simulink model "hot_region_scheduler"  (R2021a)
settings: Solver=VariableStepAuto  StartTime=0.0  StopTime=10.0  RelTol=1e-3
model workspace (MAT data in the model file):
  region_count = 6
  store_count = 4
libraries: pingcap x4
settings Model: Creator=tongjian  LastModifiedBy=tongjian

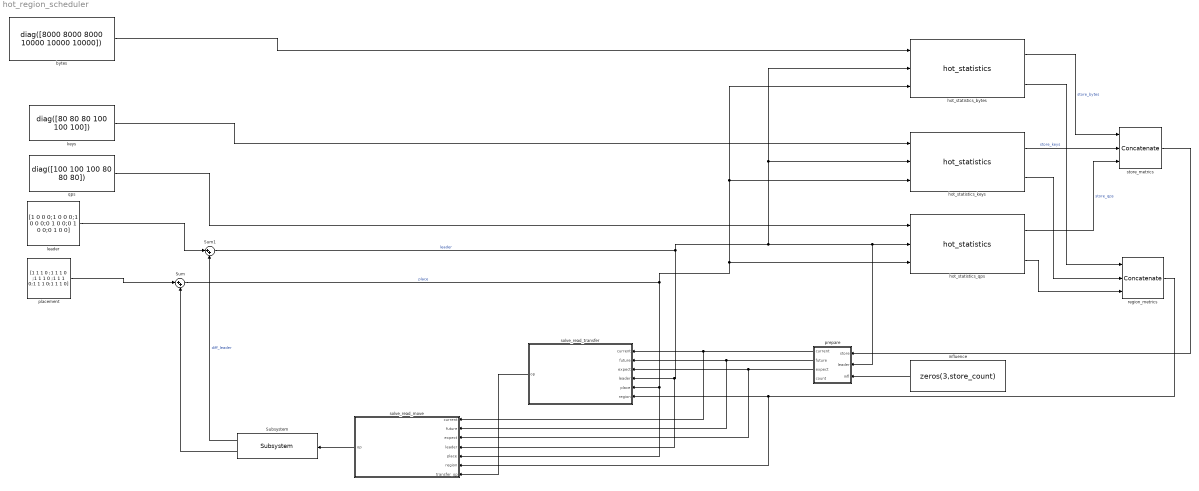
== system hot_region_scheduler ==
  Subsystem : pingcap/Subsystem  g_Ts=0.1  g_region_count=region_count  g_store_count=store_count
  Sum : Sum  Inputs=|++
  Sum1 : Sum  Inputs=|++
  bytes : Constant  Value="diag([8000 8000 8000  10000 10000 10000])"  VectorParams1D=off
  hot_statistics_bytes : pingcap/hot_statistics  g_region_dims=region_count
  hot_statistics_keys : pingcap/hot_statistics  g_region_dims=region_count
  hot_statistics_qps : pingcap/hot_statistics  g_region_dims=region_count
  influence : Constant  Value=zeros(3,store_count)  VectorParams1D=off
  keys : Constant  Value=diag([80 80 80 100 100 100])  VectorParams1D=off
  leader : Constant  Value=[1 0 0 0;1 0 0 0;1 0 0 0;0 1 0 0;0 1 0 0;0 1 0 0]  VectorParams1D=off
  placement : Constant  Value=[1 1 1 0 ;1 1 1 0 ;1 1 1 0 ;1 1 1 0;1 1 1 0;1 1 1 0]  VectorParams1D=off
  prepare : MATLAB Function  TreatAsAtomicUnit=on
  qps : Constant  Value=diag([100 100 100 80 80 80])  VectorParams1D=off
  region_metrics : Concatenate  NumInputs=3  Mode=Multidimensional array
  solve_read_move : MATLAB Function  TreatAsAtomicUnit=on
  solve_read_transfer : MATLAB Function  TreatAsAtomicUnit=on
  store_metrics : Concatenate  NumInputs=3  Mode=Multidimensional array
  wires:
  placement/1 -> Sum/1
  influence/1 -> prepare/3(infl)
  prepare/1(current) -> solve_read_move/1(current), solve_read_transfer/1(current)
  hot_statistics_bytes/1 -> store_metrics/1  "store_bytes"
  hot_statistics_keys/1 -> store_metrics/2  "store_keys"
  store_metrics/1 -> prepare/1(store)
  Sum/1 -> hot_statistics_bytes/3, hot_statistics_keys/3, hot_statistics_qps/3, solve_read_move/5(place), solve_read_transfer/5(place)  "place"
  qps/1 -> hot_statistics_qps/1
  keys/1 -> hot_statistics_keys/1
  bytes/1 -> hot_statistics_bytes/1
  leader/1 -> Sum1/1
  Sum1/1 -> hot_statistics_bytes/2, hot_statistics_keys/2, prepare/2(leader), hot_statistics_qps/2, solve_read_move/4(leader), solve_read_transfer/4(leader)  "leader"
  hot_statistics_bytes/2 -> region_metrics/1
  hot_statistics_keys/2 -> region_metrics/2
  region_metrics/1 -> solve_read_move/6(region), solve_read_transfer/6(region)
  prepare/2(future) -> solve_read_move/2(future), solve_read_transfer/2(future)
  prepare/3(expect) -> solve_read_move/3(expect), solve_read_transfer/3(expect)
  Subsystem/1 -> Sum1/2  "diff_leader"
  hot_statistics_qps/1 -> store_metrics/3  "store_qps"
  hot_statistics_qps/2 -> region_metrics/3
  Subsystem/2 -> Sum/2
  solve_read_transfer/1(op) -> solve_read_move/7(transfer_op)
  solve_read_move/1(op) -> Subsystem/1

== matlab function hot_region_scheduler/prepare ==
  data: store input; leader input; current output; future output; expect output; infl input; count output

%  计算current,future,expect
%  store dims：bytes keys query
%  count: hot region count in each store
function [current,future,expect,count]= fcn(store,leader,infl)
current=store;
%  计算store 每个维度的平均值
expect=mean(store,2);
future=current+infl;
count=sum(leader);
end

== matlab function hot_region_scheduler/solve_read_transfer ==
  data: current input; op output; future input; expect input; leader input; place input; region input
%  generator transfer operator (srcStore,desStore,regionId）
function op = fcn(current, future,expect,leader,place,region)
src_tolerance_ratio=1.05;
des_tolerator_ratio=1.05;
%  step 1: pick src ,the load must gt expect
minLoad=min(current,future);
maxLoad=max(current,future);
[n,m]=size(current);
srcs=zeros(1,m);

%  pick src store
for i=1:m
    pass=1;
    for j=1:n
        if minLoad(j,i)<expect(j)*src_tolerance_ratio
            pass=0;
            break
        end
    end
    if pass==1
        srcs(i)=1;
    end
end
op=[0,0,0,1];
rank=0;
% step 2 range src
for i=1:m
    if srcs(i)<1
        continue
    end
%     src=i;
    %  find leader region in store
    regionIds=leader(:,i);
    regionIds=find(regionIds==1);
    
    for j=1:size(regionIds,2)
%       find all region can transport exclude itself
        regionID=regionIds(j);
        
        dsts=place(regionID,:);
        dsts=find(dsts==1);
        dsts(:,i)=[];
       
        for k=1:size(dsts,2)
            storeId=dsts(k);
            load=maxLoad(:,storeId);
            for m=1:size(load,1)
                if load(m)>expect(m)*des_tolerator_ratio
                    dsts(k)=0;
                    break
                end
            end
        end
        dsts=dsts(dsts>0);
        for k=1:size(dsts,2)
            srcLd=minLoad(:,i);
            dstLd=maxLoad(:,dsts(k));
            peer=region(:,regionID);
            r=calcProgressiveRank(srcLd,dstLd,peer);
            if r<rank
                op=[i,dsts(k),regionID,1];
                rank=r;
            end
        end
    end
end
end

== matlab function hot_region_scheduler/solve_read_move ==
  data: current input; op output; future input; expect input; leader input; place input; region input; transfer_op input
%  generator transfer operator (srcStore,desStore,regionId）
function op = fcn(current, future,expect,leader,place,region,transfer_op)
if transfer_op(1)>0
    op=transfer_op;
    return 
end 
src_tolerance_ratio=1.05;
des_tolerator_ratio=1.05;
%  step 1: pick src ,the load must gt expect
minLoad=min(current,future);
maxLoad=max(current,future);
[n,m]=size(current);
srcs=zeros(1,m);

%  pick src store
for i=1:m
    pass=1;
    for j=1:n
        if minLoad(j,i)<expect(j)*src_tolerance_ratio
            pass=0;
            break
        end
    end
    if pass==1
        srcs(i)=1;
    end
end
op=[0,0,0,2];
rank=0;
% step 2 range src
for i=1:m
    if srcs(i)<1
        continue
    end
%     src=i;
    %  find leader region in store
    regionIds=leader(:,i);
    regionIds=find(regionIds==1);
    
    for j=1:size(regionIds,2)
%       find all region can transport exclude itself
        regionID=regionIds(j);
        
        dsts=place(regionID,:);
        dsts=find(dsts==0);
       
        for k=1:size(dsts,2)
            storeId=dsts(k);
            load=maxLoad(:,storeId);
            for m=1:size(load,1)
                if load(m)>expect(m)/des_tolerator_ratio
                    dsts(k)=0;
                    break
                end
            end
        end
        dsts=dsts(dsts>0);
        for k=1:size(dsts,2)
            srcLd=minLoad(:,i);
            dstLd=maxLoad(:,dsts(k));
            peer=region(:,regionID);
            r=calcProgressiveRank(srcLd,dstLd,peer);
            if r<rank
                op=[i,dsts(k),regionID,2];
                rank=r;
            end
        end
    end
end
% op=[0,0,0,2];
end
